simulink model "Drugi"  (R2015b)
settings: Solver=FixedStepAuto  StartTime=0.0  StopTime=10  FixedStep=0.01  RelTol=1e-3
undefined symbols (not defined in the file or in its folder): d, g, I, K_M, K_prop, ksi, m, T_M, x
libraries: simulink x1
settings Model: Creator=Erdal  LastModifiedBy=Erdal

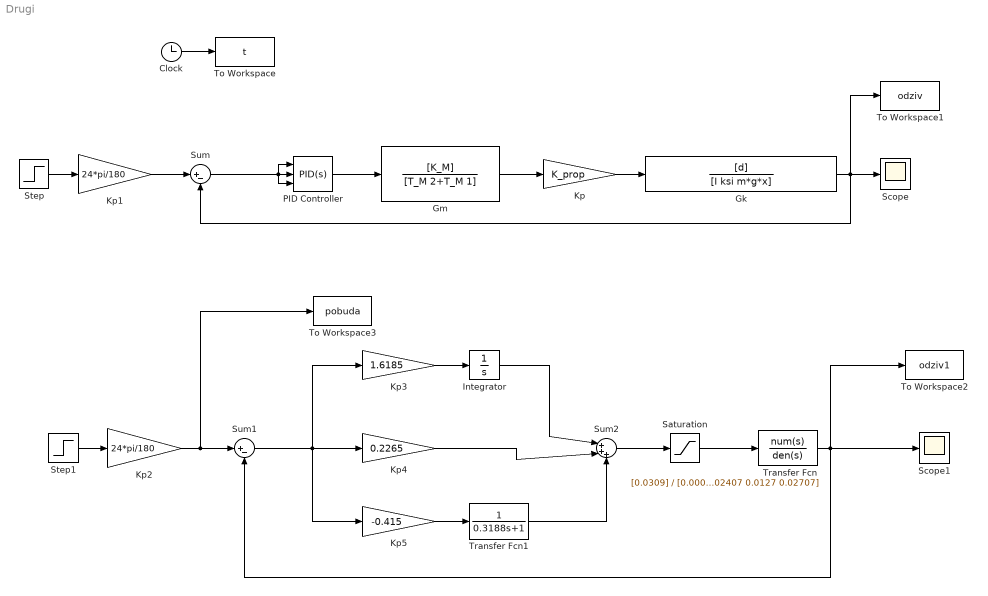
== system Drugi ==
  Clock : Clock
  Gk : TransferFcn  Numerator=[d]  Denominator=[I ksi m*g*x]
  Gm : TransferFcn  Numerator=[K_M]  Denominator=[T_M 2+T_M 1]
  Integrator : Integrator  LimitOutput=on  UpperSaturationLimit=3  LowerSaturationLimit=0
  Kp : Gain  Gain=K_prop
  Kp1 : Gain  Gain=24*pi/180
  Kp2 : Gain  Gain=24*pi/180
  Kp3 : Gain  Gain=1.6185
  Kp4 : Gain  Gain=0.2265
  Kp5 : Gain  Gain=-0.415
  PID Controller : simulink/Continuous/PID Controller  Controller=PID  TimeDomain=Continuous-time  SampleTime=-1  IntegratorMethod=Forward Euler  FilterMethod=Forward Euler  Form=Parallel  UseFilter=on  ControllerParametersSource=internal  P=1.506  I=1.132  D=-0.182  N=2.606  InitialConditionSource=external  InitialConditionForIntegrator=0  InitialConditionForFilter=0  ExternalReset=none  LimitOutput=on  UpperSaturationLimit=3  LowerSaturationLimit=0  LinearizeAsGain=on  AntiWindupMode=none  Kb=1  TrackingMode=off  Kt=1  PParamMin=[]  PParamMax=[]  IParamMin=[]  IParamMax=[]  DParamMin=[]  DParamMax=[]  NParamMin=[]  NParamMax=[]  KbParamMin=[]  KbParamMax=[]  KtParamMin=[]  KtParamMax=[]  POutMin=[]  POutMax=[]  IOutMin=[]  IOutMax=[]  DOutMin=[]  DOutMax=[]  NOutMin=[]  NOutMax=[]  KbOutMin=[]  KbOutMax=[]  KtOutMin=[]  KtOutMax=[]  IntegratorOutMin=[]  IntegratorOutMax=[]  FilterOutMin=[]  FilterOutMax=[]  SumOutMin=[]  SumOutMax=[]  SumI1OutMin=[]  SumI1OutMax=[]  SumI2OutMin=[]  SumI2OutMax=[]  SumI3OutMin=[]  SumI3OutMax=[]  SumDOutMin=[]  SumDOutMax=[]  SaturationOutMin=[]  SaturationOutMax=[]  IntegratorContinuousStateAttributes=''  IntegratorStateMustResolveToSignalObject=off  IntegratorRTWStateStorageClass=Auto  FilterContinuousStateAttributes=''  FilterStateMustResolveToSignalObject=off  FilterRTWStateStorageClass=Auto  DifferentiatorICPrevScaledInput=0  DifferentiatorOutMin=[]  DifferentiatorOutMax=[]
  Saturation : Saturate  UpperLimit=3  LowerLimit=0
  Scope : Scope
  Scope1 : Scope
  Step : Step  SampleTime=0
  Step1 : Step  SampleTime=0
  Sum : Sum  Inputs=|+-
  Sum1 : Sum  Inputs=|+-
  Sum2 : Sum  Inputs=|+++
  To Workspace : ToWorkspace  VariableName=t  SampleTime=-1
  To Workspace1 : ToWorkspace  VariableName=odziv  SampleTime=-1
  To Workspace2 : ToWorkspace  VariableName=odziv1  SampleTime=-1
  To Workspace3 : ToWorkspace  VariableName=pobuda  SampleTime=-1
  Transfer Fcn : TransferFcn  Numerator=[0.0309]  Denominator=[0.0000222 0.0003009 0.002407 0.0127 0.02707]
  Transfer Fcn1 : TransferFcn  Denominator=[0.3188 1]
  wires:
  Gm/1 -> Kp/1
  Kp/1 -> Gk/1
  PID Controller/1 -> Gm/1
  Step/1 -> Kp1/1
  Kp1/1 -> Sum/1
  Gk/1 -> To Workspace1/1, Sum/2, Scope/1
  Sum/1 -> PID Controller/3, PID Controller/2, PID Controller/1
  Clock/1 -> To Workspace/1
  Step1/1 -> Kp2/1
  Kp2/1 -> To Workspace3/1, Sum1/1
  Sum1/1 -> Kp5/1, Kp3/1, Kp4/1
  Kp3/1 -> Integrator/1
  Kp5/1 -> Transfer Fcn1/1
  Integrator/1 -> Sum2/1
  Kp4/1 -> Sum2/2
  Sum2/1 -> Saturation/1
  Saturation/1 -> Transfer Fcn/1
  Transfer Fcn/1 -> To Workspace2/1, Sum1/2, Scope1/1
  Transfer Fcn1/1 -> Sum2/3
